simulink model "parallel_prediction_and_cost_function_6phase"  (R2022a)
settings: Solver=FixedStepDiscrete  StartTime=0.0  StopTime=10.0  RelTol=1e-3
undefined symbols (not defined in the file or in its folder): f_c, L_d, L_q, L_x, L_y, p, psi_pm, R_ph
libraries: hdlsllib x5
(part 2 of 3)

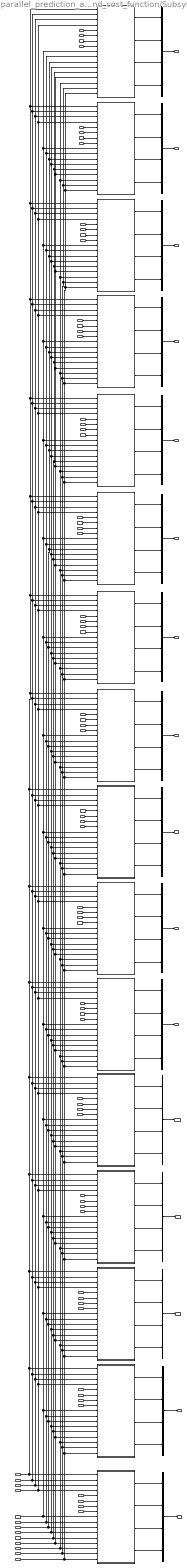
== system parallel_prediction_and_cost_function_6phase/Prediction_and_cost_function/Subsystem ==
  d_phase_voltage_per_switching_state : Inport
  q_phase_voltage_per_switching_state : Inport  Port=2
  x_phase_voltage_per_switching_state : Inport  Port=3
  y_phase_voltage_per_switching_state : Inport  Port=4
  d_phase_voltage_per_switching_state1 : Inport  Port=5
  q_phase_voltage_per_switching_state1 : Inport  Port=6
  x_phase_voltage_per_switching_state1 : Inport  Port=7
  y_phase_voltage_per_switching_state1 : Inport  Port=8
  d_phase_voltage_per_switching_state2 : Inport  Port=9
  q_phase_voltage_per_switching_state2 : Inport  Port=10
  x_phase_voltage_per_switching_state2 : Inport  Port=11
  y_phase_voltage_per_switching_state2 : Inport  Port=12
  d_phase_voltage_per_switching_state3 : Inport  Port=13
  q_phase_voltage_per_switching_state3 : Inport  Port=14
  x_phase_voltage_per_switching_state3 : Inport  Port=15
  y_phase_voltage_per_switching_state3 : Inport  Port=16
  d_phase_voltage_per_switching_state4 : Inport  Port=17
  q_phase_voltage_per_switching_state4 : Inport  Port=18
  x_phase_voltage_per_switching_state4 : Inport  Port=19
  y_phase_voltage_per_switching_state4 : Inport  Port=20
  d_phase_voltage_per_switching_state5 : Inport  Port=21
  q_phase_voltage_per_switching_state5 : Inport  Port=22
  x_phase_voltage_per_switching_state5 : Inport  Port=23
  y_phase_voltage_per_switching_state5 : Inport  Port=24
  d_phase_voltage_per_switching_state6 : Inport  Port=25
  q_phase_voltage_per_switching_state6 : Inport  Port=26
  x_phase_voltage_per_switching_state6 : Inport  Port=27
  y_phase_voltage_per_switching_state6 : Inport  Port=28
  d_phase_voltage_per_switching_state7 : Inport  Port=29
  q_phase_voltage_per_switching_state7 : Inport  Port=30
  x_phase_voltage_per_switching_state7 : Inport  Port=31
  y_phase_voltage_per_switching_state7 : Inport  Port=32
  d_phase_voltage_per_switching_state8 : Inport  Port=33
  q_phase_voltage_per_switching_state8 : Inport  Port=34
  x_phase_voltage_per_switching_state8 : Inport  Port=35
  y_phase_voltage_per_switching_state8 : Inport  Port=36
  d_phase_voltage_per_switching_state9 : Inport  Port=37
  q_phase_voltage_per_switching_state9 : Inport  Port=38
  x_phase_voltage_per_switching_state9 : Inport  Port=39
  y_phase_voltage_per_switching_state9 : Inport  Port=40
  d_phase_voltage_per_switching_state10 : Inport  Port=41
  q_phase_voltage_per_switching_state10 : Inport  Port=42
  x_phase_voltage_per_switching_state10 : Inport  Port=43
  y_phase_voltage_per_switching_state10 : Inport  Port=44
  d_phase_voltage_per_switching_state11 : Inport  Port=45
  q_phase_voltage_per_switching_state11 : Inport  Port=46
  x_phase_voltage_per_switching_state11 : Inport  Port=47
  y_phase_voltage_per_switching_state11 : Inport  Port=48
  d_phase_voltage_per_switching_state12 : Inport  Port=49
  q_phase_voltage_per_switching_state12 : Inport  Port=50
  x_phase_voltage_per_switching_state12 : Inport  Port=51
  y_phase_voltage_per_switching_state12 : Inport  Port=52
  d_phase_voltage_per_switching_state13 : Inport  Port=53
  q_phase_voltage_per_switching_state13 : Inport  Port=54
  x_phase_voltage_per_switching_state13 : Inport  Port=55
  y_phase_voltage_per_switching_state13 : Inport  Port=56
  d_phase_voltage_per_switching_state14 : Inport  Port=57
  q_phase_voltage_per_switching_state14 : Inport  Port=58
  x_phase_voltage_per_switching_state14 : Inport  Port=59
  y_phase_voltage_per_switching_state14 : Inport  Port=60
  SampleTime_div_Ld15 : Inport  Port=61
  SampleTime_div_Lq15 : Inport  Port=62
  SampleTime_div_Lx15 : Inport  Port=63
  SampleTime_div_Ly15 : Inport  Port=64
  id_k_16 : Inport  Port=65
  iq_k_16 : Inport  Port=66
  ix_k_16 : Inport  Port=67
  iy_k_16 : Inport  Port=68
  Rs15 : Inport  Port=69
  omega_el15 : Inport  Port=70
  Lq15 : Inport  Port=71
  Ld15 : Inport  Port=72
  psiPM15 : Inport  Port=73
  d_phase_voltage_per_switching_state15 : Inport  Port=74
  q_phase_voltage_per_switching_state15 : Inport  Port=75
  x_phase_voltage_per_switching_state15 : Inport  Port=76
  y_phase_voltage_per_switching_state15 : Inport  Port=77
  Mux{,1..15} (16 alike) : Mux
  Subsystem : Subsystem
  Subsystem1 : Subsystem
  Subsystem10 : Subsystem
  Subsystem11 : Subsystem
  Subsystem12 : Subsystem
  Subsystem13 : Subsystem
  Subsystem14 : Subsystem
  Subsystem15 : Subsystem
  Subsystem2 : Subsystem
  Subsystem3 : Subsystem
  Subsystem4 : Subsystem
  Subsystem5 : Subsystem
  Subsystem6 : Subsystem
  Subsystem7 : Subsystem
  Subsystem8 : Subsystem
  Subsystem9 : Subsystem
  Prediction_1 : Outport
  Prediction_2 : Outport  Port=2
  Prediction_3 : Outport  Port=3
  Prediction_4 : Outport  Port=4
  Prediction_5 : Outport  Port=5
  Prediction_6 : Outport  Port=6
  Prediction_7 : Outport  Port=7
  Prediction_8 : Outport  Port=8
  Prediction_9 : Outport  Port=9
  Prediction_10 : Outport  Port=10
  Prediction_11 : Outport  Port=11
  Prediction_12 : Outport  Port=12
  Prediction_13 : Outport  Port=13
  Prediction_14 : Outport  Port=14
  Prediction_15 : Outport  Port=15
  Prediction_16 : Outport  Port=16
  wires:
  d_phase_voltage_per_switching_state13/1 -> Subsystem2/5(d_phase_voltage_per_switching_state)
  q_phase_voltage_per_switching_state1/1 -> Subsystem14/6(q_phase_voltage_per_switching_state)
  x_phase_voltage_per_switching_state12/1 -> Subsystem3/7(x_phase_voltage_per_switching_state)
  y_phase_voltage_per_switching_state/1 -> Subsystem15/8(y_phase_voltage_per_switching_state)
  y_phase_voltage_per_switching_state2/1 -> Subsystem13/8(y_phase_voltage_per_switching_state)
  d_phase_voltage_per_switching_state1/1 -> Subsystem14/5(d_phase_voltage_per_switching_state)
  x_phase_voltage_per_switching_state1/1 -> Subsystem14/7(x_phase_voltage_per_switching_state)
  y_phase_voltage_per_switching_state7/1 -> Subsystem8/8(y_phase_voltage_per_switching_state)
  d_phase_voltage_per_switching_state3/1 -> Subsystem12/5(d_phase_voltage_per_switching_state)
  d_phase_voltage_per_switching_state6/1 -> Subsystem9/5(d_phase_voltage_per_switching_state)
  x_phase_voltage_per_switching_state9/1 -> Subsystem6/7(x_phase_voltage_per_switching_state)
  d_phase_voltage_per_switching_state/1 -> Subsystem15/5(d_phase_voltage_per_switching_state)
  x_phase_voltage_per_switching_state3/1 -> Subsystem12/7(x_phase_voltage_per_switching_state)
  d_phase_voltage_per_switching_state2/1 -> Subsystem13/5(d_phase_voltage_per_switching_state)
  x_phase_voltage_per_switching_state8/1 -> Subsystem7/7(x_phase_voltage_per_switching_state)
  y_phase_voltage_per_switching_state9/1 -> Subsystem6/8(y_phase_voltage_per_switching_state)
  x_phase_voltage_per_switching_state4/1 -> Subsystem11/7(x_phase_voltage_per_switching_state)
  y_phase_voltage_per_switching_state1/1 -> Subsystem14/8(y_phase_voltage_per_switching_state)
  q_phase_voltage_per_switching_state2/1 -> Subsystem13/6(q_phase_voltage_per_switching_state)
  x_phase_voltage_per_switching_state2/1 -> Subsystem13/7(x_phase_voltage_per_switching_state)
  y_phase_voltage_per_switching_state11/1 -> Subsystem4/8(y_phase_voltage_per_switching_state)
  y_phase_voltage_per_switching_state4/1 -> Subsystem11/8(y_phase_voltage_per_switching_state)
  x_phase_voltage_per_switching_state/1 -> Subsystem15/7(x_phase_voltage_per_switching_state)
  d_phase_voltage_per_switching_state14/1 -> Subsystem1/5(d_phase_voltage_per_switching_state)
  q_phase_voltage_per_switching_state9/1 -> Subsystem6/6(q_phase_voltage_per_switching_state)
  q_phase_voltage_per_switching_state5/1 -> Subsystem10/6(q_phase_voltage_per_switching_state)
  d_phase_voltage_per_switching_state10/1 -> Subsystem5/5(d_phase_voltage_per_switching_state)
  x_phase_voltage_per_switching_state14/1 -> Subsystem1/7(x_phase_voltage_per_switching_state)
  y_phase_voltage_per_switching_state14/1 -> Subsystem1/8(y_phase_voltage_per_switching_state)
  q_phase_voltage_per_switching_state14/1 -> Subsystem1/6(q_phase_voltage_per_switching_state)
  q_phase_voltage_per_switching_state11/1 -> Subsystem4/6(q_phase_voltage_per_switching_state)
  x_phase_voltage_per_switching_state11/1 -> Subsystem4/7(x_phase_voltage_per_switching_state)
  d_phase_voltage_per_switching_state11/1 -> Subsystem4/5(d_phase_voltage_per_switching_state)
  y_phase_voltage_per_switching_state12/1 -> Subsystem3/8(y_phase_voltage_per_switching_state)
  x_phase_voltage_per_switching_state13/1 -> Subsystem2/7(x_phase_voltage_per_switching_state)
  d_phase_voltage_per_switching_state9/1 -> Subsystem6/5(d_phase_voltage_per_switching_state)
  d_phase_voltage_per_switching_state7/1 -> Subsystem8/5(d_phase_voltage_per_switching_state)
  d_phase_voltage_per_switching_state4/1 -> Subsystem11/5(d_phase_voltage_per_switching_state)
  q_phase_voltage_per_switching_state4/1 -> Subsystem11/6(q_phase_voltage_per_switching_state)
  q_phase_voltage_per_switching_state12/1 -> Subsystem3/6(q_phase_voltage_per_switching_state)
  d_phase_voltage_per_switching_state8/1 -> Subsystem7/5(d_phase_voltage_per_switching_state)
  x_phase_voltage_per_switching_state5/1 -> Subsystem10/7(x_phase_voltage_per_switching_state)
  d_phase_voltage_per_switching_state12/1 -> Subsystem3/5(d_phase_voltage_per_switching_state)
  x_phase_voltage_per_switching_state7/1 -> Subsystem8/7(x_phase_voltage_per_switching_state)
  q_phase_voltage_per_switching_state/1 -> Subsystem15/6(q_phase_voltage_per_switching_state)
  d_phase_voltage_per_switching_state5/1 -> Subsystem10/5(d_phase_voltage_per_switching_state)
  q_phase_voltage_per_switching_state13/1 -> Subsystem2/6(q_phase_voltage_per_switching_state)
  y_phase_voltage_per_switching_state5/1 -> Subsystem10/8(y_phase_voltage_per_switching_state)
  q_phase_voltage_per_switching_state6/1 -> Subsystem9/6(q_phase_voltage_per_switching_state)
  y_phase_voltage_per_switching_state6/1 -> Subsystem9/8(y_phase_voltage_per_switching_state)
  x_phase_voltage_per_switching_state6/1 -> Subsystem9/7(x_phase_voltage_per_switching_state)
  y_phase_voltage_per_switching_state8/1 -> Subsystem7/8(y_phase_voltage_per_switching_state)
  q_phase_voltage_per_switching_state8/1 -> Subsystem7/6(q_phase_voltage_per_switching_state)
  y_phase_voltage_per_switching_state13/1 -> Subsystem2/8(y_phase_voltage_per_switching_state)
  q_phase_voltage_per_switching_state7/1 -> Subsystem8/6(q_phase_voltage_per_switching_state)
  x_phase_voltage_per_switching_state10/1 -> Subsystem5/7(x_phase_voltage_per_switching_state)
  q_phase_voltage_per_switching_state10/1 -> Subsystem5/6(q_phase_voltage_per_switching_state)
  y_phase_voltage_per_switching_state10/1 -> Subsystem5/8(y_phase_voltage_per_switching_state)
  y_phase_voltage_per_switching_state3/1 -> Subsystem12/8(y_phase_voltage_per_switching_state)
  q_phase_voltage_per_switching_state3/1 -> Subsystem12/6(q_phase_voltage_per_switching_state)
  SampleTime_div_Ld15/1 -> Subsystem/1(SampleTime_div_Ld), Subsystem4/1(SampleTime_div_Ld), Subsystem7/1(SampleTime_div_Ld), Subsystem15/1(SampleTime_div_Ld), Subsystem14/1(SampleTime_div_Ld), Subsystem13/1(SampleTime_div_Ld), Subsystem12/1(SampleTime_div_Ld), Subsystem11/1(SampleTime_div_Ld), Subsystem10/1(SampleTime_div_Ld), Subsystem9/1(SampleTime_div_Ld), Subsystem8/1(SampleTime_div_Ld), Subsystem6/1(SampleTime_div_Ld), Subsystem5/1(SampleTime_div_Ld), Subsystem3/1(SampleTime_div_Ld), Subsystem2/1(SampleTime_div_Ld), Subsystem1/1(SampleTime_div_Ld)  "SampleTime_div_Ld"
  SampleTime_div_Lq15/1 -> Subsystem/2(SampleTime_div_Lq), Subsystem4/2(SampleTime_div_Lq), Subsystem15/2(SampleTime_div_Lq), Subsystem14/2(SampleTime_div_Lq), Subsystem13/2(SampleTime_div_Lq), Subsystem12/2(SampleTime_div_Lq), Subsystem11/2(SampleTime_div_Lq), Subsystem10/2(SampleTime_div_Lq), Subsystem9/2(SampleTime_div_Lq), Subsystem8/2(SampleTime_div_Lq), Subsystem7/2(SampleTime_div_Lq), Subsystem6/2(SampleTime_div_Lq), Subsystem5/2(SampleTime_div_Lq), Subsystem3/2(SampleTime_div_Lq), Subsystem2/2(SampleTime_div_Lq), Subsystem1/2(SampleTime_div_Lq)  "SampleTime_div_Lq"
  SampleTime_div_Lx15/1 -> Subsystem/3(SampleTime_div_Lx), Subsystem15/3(SampleTime_div_Lx), Subsystem14/3(SampleTime_div_Lx), Subsystem13/3(SampleTime_div_Lx), Subsystem12/3(SampleTime_div_Lx), Subsystem11/3(SampleTime_div_Lx), Subsystem10/3(SampleTime_div_Lx), Subsystem9/3(SampleTime_div_Lx), Subsystem8/3(SampleTime_div_Lx), Subsystem7/3(SampleTime_div_Lx), Subsystem6/3(SampleTime_div_Lx), Subsystem5/3(SampleTime_div_Lx), Subsystem4/3(SampleTime_div_Lx), Subsystem3/3(SampleTime_div_Lx), Subsystem2/3(SampleTime_div_Lx), Subsystem1/3(SampleTime_div_Lx)  "SampleTime_div_Lx"
  SampleTime_div_Ly15/1 -> Subsystem15/4(SampleTime_div_Ly), Subsystem14/4(SampleTime_div_Ly), Subsystem13/4(SampleTime_div_Ly), Subsystem12/4(SampleTime_div_Ly), Subsystem11/4(SampleTime_div_Ly), Subsystem10/4(SampleTime_div_Ly), Subsystem9/4(SampleTime_div_Ly), Subsystem8/4(SampleTime_div_Ly), Subsystem7/4(SampleTime_div_Ly), Subsystem6/4(SampleTime_div_Ly), Subsystem5/4(SampleTime_div_Ly), Subsystem4/4(SampleTime_div_Ly), Subsystem3/4(SampleTime_div_Ly), Subsystem2/4(SampleTime_div_Ly), Subsystem1/4(SampleTime_div_Ly), Subsystem/4(SampleTime_div_Ly)  "SampleTime_div_Ly"
  d_phase_voltage_per_switching_state15/1 -> Subsystem/5(d_phase_voltage_per_switching_state)
  q_phase_voltage_per_switching_state15/1 -> Subsystem/6(q_phase_voltage_per_switching_state)
  x_phase_voltage_per_switching_state15/1 -> Subsystem/7(x_phase_voltage_per_switching_state)
  y_phase_voltage_per_switching_state15/1 -> Subsystem/8(y_phase_voltage_per_switching_state)
  id_k_16/1 -> Subsystem/9(id_k), Subsystem15/9(id_k), Subsystem14/9(id_k), Subsystem13/9(id_k), Subsystem12/9(id_k), Subsystem11/9(id_k), Subsystem10/9(id_k), Subsystem9/9(id_k), Subsystem8/9(id_k), Subsystem7/9(id_k), Subsystem6/9(id_k), Subsystem5/9(id_k), Subsystem4/9(id_k), Subsystem3/9(id_k), Subsystem2/9(id_k), Subsystem1/9(id_k)  "id_k"
  iq_k_16/1 -> Subsystem/10(iq_k), Subsystem15/10(iq_k), Subsystem14/10(iq_k), Subsystem13/10(iq_k), Subsystem12/10(iq_k), Subsystem11/10(iq_k), Subsystem10/10(iq_k), Subsystem9/10(iq_k), Subsystem8/10(iq_k), Subsystem7/10(iq_k), Subsystem6/10(iq_k), Subsystem5/10(iq_k), Subsystem4/10(iq_k), Subsystem3/10(iq_k), Subsystem2/10(iq_k), Subsystem1/10(iq_k)  "iq_k"
  ix_k_16/1 -> Subsystem/11(ix_k), Subsystem15/11(ix_k), Subsystem14/11(ix_k), Subsystem13/11(ix_k), Subsystem12/11(ix_k), Subsystem11/11(ix_k), Subsystem10/11(ix_k), Subsystem9/11(ix_k), Subsystem8/11(ix_k), Subsystem7/11(ix_k), Subsystem6/11(ix_k), Subsystem5/11(ix_k), Subsystem4/11(ix_k), Subsystem3/11(ix_k), Subsystem2/11(ix_k), Subsystem1/11(ix_k)  "ix_k"
  iy_k_16/1 -> Subsystem/12(iy_k), Subsystem15/12(iy_k), Subsystem14/12(iy_k), Subsystem13/12(iy_k), Subsystem12/12(iy_k), Subsystem11/12(iy_k), Subsystem10/12(iy_k), Subsystem9/12(iy_k), Subsystem8/12(iy_k), Subsystem7/12(iy_k), Subsystem6/12(iy_k), Subsystem5/12(iy_k), Subsystem4/12(iy_k), Subsystem3/12(iy_k), Subsystem2/12(iy_k), Subsystem1/12(iy_k)  "iy_k"
  psiPM15/1 -> Subsystem/13(psiPM), Subsystem10/13(psiPM), Subsystem15/13(psiPM), Subsystem14/13(psiPM), Subsystem13/13(psiPM), Subsystem12/13(psiPM), Subsystem11/13(psiPM), Subsystem9/13(psiPM), Subsystem8/13(psiPM), Subsystem7/13(psiPM), Subsystem6/13(psiPM), Subsystem5/13(psiPM), Subsystem4/13(psiPM), Subsystem3/13(psiPM), Subsystem2/13(psiPM), Subsystem1/13(psiPM)  "psiPM"
  Lq15/1 -> Subsystem/14(Lq), Subsystem15/14(Lq), Subsystem14/14(Lq), Subsystem13/14(Lq), Subsystem12/14(Lq), Subsystem11/14(Lq), Subsystem10/14(Lq), Subsystem9/14(Lq), Subsystem8/14(Lq), Subsystem7/14(Lq), Subsystem6/14(Lq), Subsystem5/14(Lq), Subsystem4/14(Lq), Subsystem3/14(Lq), Subsystem2/14(Lq), Subsystem1/14(Lq)  "Lq"
  Ld15/1 -> Subsystem/15(Ld), Subsystem1/15(Ld), Subsystem15/15(Ld), Subsystem14/15(Ld), Subsystem13/15(Ld), Subsystem12/15(Ld), Subsystem11/15(Ld), Subsystem10/15(Ld), Subsystem9/15(Ld), Subsystem8/15(Ld), Subsystem7/15(Ld), Subsystem6/15(Ld), Subsystem5/15(Ld), Subsystem4/15(Ld), Subsystem3/15(Ld), Subsystem2/15(Ld)  "Ld"
  Rs15/1 -> Subsystem/16(Rs), Subsystem7/16(Rs), Subsystem15/16(Rs), Subsystem14/16(Rs), Subsystem13/16(Rs), Subsystem12/16(Rs), Subsystem11/16(Rs), Subsystem10/16(Rs), Subsystem9/16(Rs), Subsystem8/16(Rs), Subsystem6/16(Rs), Subsystem5/16(Rs), Subsystem4/16(Rs), Subsystem3/16(Rs), Subsystem2/16(Rs), Subsystem1/16(Rs)  "Rs"
  omega_el15/1 -> Subsystem/17(omega_el), Subsystem15/17(omega_el), Subsystem14/17(omega_el), Subsystem13/17(omega_el), Subsystem12/17(omega_el), Subsystem11/17(omega_el), Subsystem10/17(omega_el), Subsystem9/17(omega_el), Subsystem8/17(omega_el), Subsystem7/17(omega_el), Subsystem6/17(omega_el), Subsystem5/17(omega_el), Subsystem4/17(omega_el), Subsystem3/17(omega_el), Subsystem2/17(omega_el), Subsystem1/17(omega_el)  "omega_el"
  Subsystem/4(iy_16) -> Mux/4
  Subsystem/3(ix_16) -> Mux/3
  Subsystem/2(iq_16) -> Mux/2
  Subsystem/1(id_16) -> Mux/1
  Mux/1 -> Prediction_16/1
  Subsystem1/2(iq_15) -> Mux1/2
  Subsystem1/3(ix_15) -> Mux1/3
  Subsystem1/1(id_15) -> Mux1/1
  Mux1/1 -> Prediction_15/1
  Subsystem1/4(iy_15) -> Mux1/4
  Subsystem2/2(iq_14) -> Mux2/2
  Subsystem2/1(id_14) -> Mux2/1
  Subsystem2/3(ix_14) -> Mux2/3
  Subsystem2/4(iy_14) -> Mux2/4
  Mux2/1 -> Prediction_14/1
  Mux3/1 -> Prediction_13/1
  Subsystem3/3(ix_13) -> Mux3/3
  Subsystem3/2(iq_13) -> Mux3/2
  Subsystem3/1(id_13) -> Mux3/1
  Subsystem3/4(iy_13) -> Mux3/4
  Subsystem4/2(iq_12) -> Mux4/2
  Subsystem4/1(id_12) -> Mux4/1
  Mux4/1 -> Prediction_12/1
  Subsystem4/4(iy_12) -> Mux4/4
  Subsystem4/3(ix_12) -> Mux4/3
  Subsystem5/2(iq_11) -> Mux5/2
  Subsystem5/3(ix_11) -> Mux5/3
  Subsystem5/1(id_11) -> Mux5/1
  Subsystem5/4(iy_11) -> Mux5/4
  Mux5/1 -> Prediction_11/1
  Subsystem6/1(id_10) -> Mux6/1
  Subsystem6/2(iq_10) -> Mux6/2
  Subsystem6/3(ix_10) -> Mux6/3
  Subsystem6/4(iy_10) -> Mux6/4
  Mux6/1 -> Prediction_10/1
  Subsystem7/3(ix_9) -> Mux7/3
  Mux7/1 -> Prediction_9/1
  Subsystem7/1(id_9) -> Mux7/1
  Subsystem7/2(iq_9) -> Mux7/2
  Subsystem7/4(iy_9) -> Mux7/4
  Subsystem8/1(id_8) -> Mux8/1
  Subsystem8/3(ix_8) -> Mux8/3
  Subsystem8/2(iq_8) -> Mux8/2
  Subsystem8/4(iy_8) -> Mux8/4
  Mux8/1 -> Prediction_8/1
  Subsystem9/1(id_7) -> Mux9/1
  Subsystem9/3(ix_7) -> Mux9/3
  Subsystem9/4(iy_7) -> Mux9/4
  Subsystem9/2(iq_7) -> Mux9/2
  Mux9/1 -> Prediction_7/1
  Subsystem10/4(iy_6) -> Mux10/4
  Subsystem10/2(iq_6) -> Mux10/2
  Subsystem10/3(ix_6) -> Mux10/3
  Subsystem10/1(id_6) -> Mux10/1
  Mux10/1 -> Prediction_6/1
  Subsystem11/3(ix_5) -> Mux11/3
  Subsystem11/4(iy_5) -> Mux11/4
  Subsystem11/2(iq_5) -> Mux11/2
  Subsystem11/1(id_5) -> Mux11/1
  Mux11/1 -> Prediction_5/1
  Subsystem12/4(iy_4) -> Mux12/4
  Subsystem12/2(iq_4) -> Mux12/2
  Mux12/1 -> Prediction_4/1
  Subsystem12/3(ix_4) -> Mux12/3
  Subsystem12/1(id_4) -> Mux12/1
  Subsystem13/2(iq_3) -> Mux13/2
  Subsystem13/4(iy_3) -> Mux13/4
  Subsystem13/3(ix_3) -> Mux13/3
  Subsystem13/1(id_3) -> Mux13/1
  Mux13/1 -> Prediction_3/1
  Subsystem14/1(id_2) -> Mux14/1
  Subsystem14/3(ix_2) -> Mux14/3
  Subsystem14/2(iq_2) -> Mux14/2
  Subsystem14/4(iy_2) -> Mux14/4
  Mux14/1 -> Prediction_2/1
  Subsystem15/4(iy_1) -> Mux15/4
  Subsystem15/2(iq_1) -> Mux15/2
  Subsystem15/1(id_1) -> Mux15/1
  Subsystem15/3(ix_1) -> Mux15/3
  Mux15/1 -> Prediction_1/1

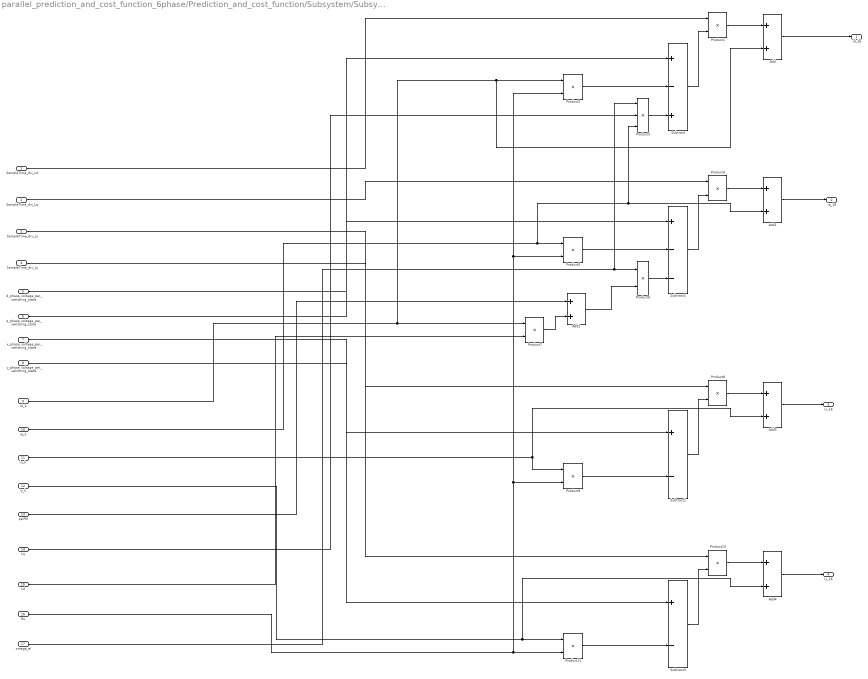
== system parallel_prediction_and_cost_function_6phase/Prediction_and_cost_function/Subsystem/Subsystem ==
  SampleTime_div_Ld : Inport
  SampleTime_div_Lq : Inport  Port=2
  SampleTime_div_Lx : Inport  Port=3
  SampleTime_div_Ly : Inport  Port=4
  d_phase_voltage_per_switching_state : Inport  Port=5
  q_phase_voltage_per_switching_state : Inport  Port=6
  x_phase_voltage_per_switching_state : Inport  Port=7
  y_phase_voltage_per_switching_state : Inport  Port=8
  id_k : Inport  Port=9
  iq_k : Inport  Port=10
  ix_k : Inport  Port=11
  iy_k : Inport  Port=12
  psiPM : Inport  Port=13
  Lq : Inport  Port=14
  Ld : Inport  Port=15
  Rs : Inport  Port=16
  omega_el : Inport  Port=17
  Add{,1,3..4} (4 alike) : Sum  OutDataTypeStr=single
  Add2 : Sum
  Product{1..2,4..11} (10 alike) : Product  OutDataTypeStr=single
  Product3 : Product  Inputs=3  OutDataTypeStr=single
  Subtract : Sum  Inputs=+-+  OutDataTypeStr=single
  Subtract1 : Sum  Inputs=+--  OutDataTypeStr=single
  Subtract2 : Sum  Inputs=+-  OutDataTypeStr=single
  Subtract3 : Sum  Inputs=+-  OutDataTypeStr=single
  id_16 : Outport
  iq_16 : Outport  Port=2
  ix_16 : Outport  Port=3
  iy_16 : Outport  Port=4
  wires:
  q_phase_voltage_per_switching_state/1 -> Subtract1/1
  omega_el/1 -> Product3/1, Product6/1
  Product5/1 -> Subtract1/2
  iq_k/1 -> Product3/3, Add1/2, Product5/1
  iy_k/1 -> Add4/2, Product11/1
  Add2/1 -> Product6/2
  Lq/1 -> Product3/2
  Subtract2/1 -> Product8/2
  SampleTime_div_Ly/1 -> Product10/1
  Rs/1 -> Product9/2, Product2/2, Product5/2, Product11/2
  Product9/1 -> Subtract2/2
  Product8/1 -> Add3/1
  Product7/1 -> Add2/2
  id_k/1 -> Add/2, Product2/1, Product7/1
  x_phase_voltage_per_switching_state/1 -> Subtract2/1
  Product11/1 -> Subtract3/2
  Product6/1 -> Subtract1/3
  Subtract1/1 -> Product4/2
  Product1/1 -> Add/1
  Product10/1 -> Add4/1
  Product4/1 -> Add1/1
  SampleTime_div_Ld/1 -> Product1/1
  y_phase_voltage_per_switching_state/1 -> Subtract3/1
  Product2/1 -> Subtract/2
  Product3/1 -> Subtract/3
  SampleTime_div_Lq/1 -> Product4/1
  Subtract/1 -> Product1/2
  Subtract3/1 -> Product10/2
  psiPM/1 -> Add2/1
  Ld/1 -> Product7/2
  ix_k/1 -> Add3/2, Product9/1
  SampleTime_div_Lx/1 -> Product8/1
  d_phase_voltage_per_switching_state/1 -> Subtract/1
  Add/1 -> id_16/1
  Add1/1 -> iq_16/1
  Add3/1 -> ix_16/1
  Add4/1 -> iy_16/1

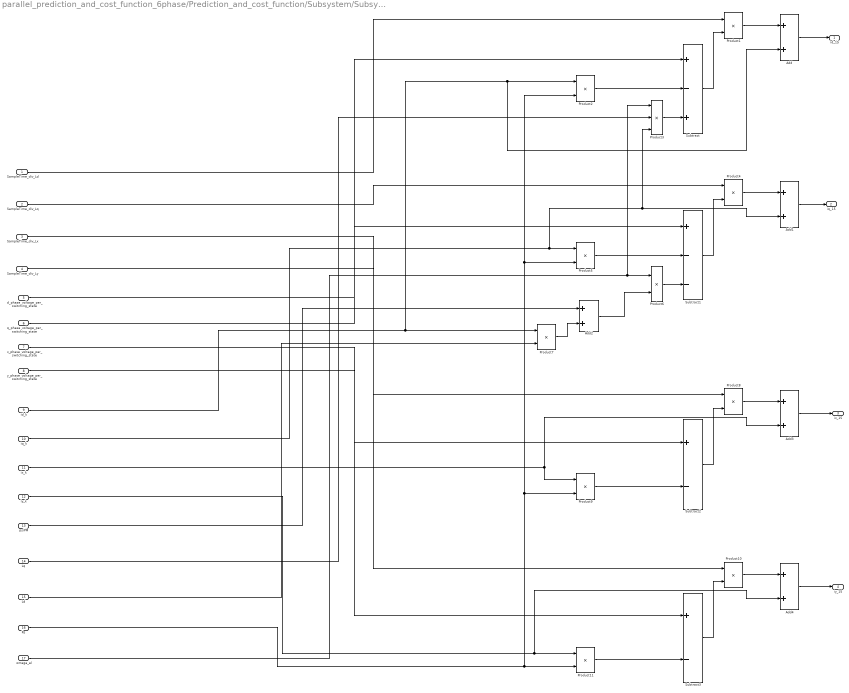
== system parallel_prediction_and_cost_function_6phase/Prediction_and_cost_function/Subsystem/Subsystem1 ==
  SampleTime_div_Ld : Inport
  SampleTime_div_Lq : Inport  Port=2
  SampleTime_div_Lx : Inport  Port=3
  SampleTime_div_Ly : Inport  Port=4
  d_phase_voltage_per_switching_state : Inport  Port=5
  q_phase_voltage_per_switching_state : Inport  Port=6
  x_phase_voltage_per_switching_state : Inport  Port=7
  y_phase_voltage_per_switching_state : Inport  Port=8
  id_k : Inport  Port=9
  iq_k : Inport  Port=10
  ix_k : Inport  Port=11
  iy_k : Inport  Port=12
  psiPM : Inport  Port=13
  Lq : Inport  Port=14
  Ld : Inport  Port=15
  Rs : Inport  Port=16
  omega_el : Inport  Port=17
  Add{,1,3..4} (4 alike) : Sum  OutDataTypeStr=single
  Add2 : Sum
  Product{1..2,4..11} (10 alike) : Product  OutDataTypeStr=single
  Product3 : Product  Inputs=3  OutDataTypeStr=single
  Subtract : Sum  Inputs=+-+  OutDataTypeStr=single
  Subtract1 : Sum  Inputs=+--  OutDataTypeStr=single
  Subtract2 : Sum  Inputs=+-  OutDataTypeStr=single
  Subtract3 : Sum  Inputs=+-  OutDataTypeStr=single
  id_15 : Outport
  iq_15 : Outport  Port=2
  ix_15 : Outport  Port=3
  iy_15 : Outport  Port=4
  wires:
  q_phase_voltage_per_switching_state/1 -> Subtract1/1
  omega_el/1 -> Product3/1, Product6/1
  Product5/1 -> Subtract1/2
  iq_k/1 -> Product3/3, Add1/2, Product5/1
  iy_k/1 -> Add4/2, Product11/1
  Add2/1 -> Product6/2
  Lq/1 -> Product3/2
  Subtract2/1 -> Product8/2
  SampleTime_div_Ly/1 -> Product10/1
  Rs/1 -> Product9/2, Product2/2, Product5/2, Product11/2
  Product9/1 -> Subtract2/2
  Product8/1 -> Add3/1
  Product7/1 -> Add2/2
  id_k/1 -> Add/2, Product2/1, Product7/1
  x_phase_voltage_per_switching_state/1 -> Subtract2/1
  Product11/1 -> Subtract3/2
  Product6/1 -> Subtract1/3
  Subtract1/1 -> Product4/2
  Product1/1 -> Add/1
  Product10/1 -> Add4/1
  Product4/1 -> Add1/1
  SampleTime_div_Ld/1 -> Product1/1
  y_phase_voltage_per_switching_state/1 -> Subtract3/1
  Product2/1 -> Subtract/2
  Product3/1 -> Subtract/3
  SampleTime_div_Lq/1 -> Product4/1
  Subtract/1 -> Product1/2
  Subtract3/1 -> Product10/2
  psiPM/1 -> Add2/1
  Ld/1 -> Product7/2
  ix_k/1 -> Add3/2, Product9/1
  SampleTime_div_Lx/1 -> Product8/1
  d_phase_voltage_per_switching_state/1 -> Subtract/1
  Add/1 -> id_15/1
  Add1/1 -> iq_15/1
  Add3/1 -> ix_15/1
  Add4/1 -> iy_15/1

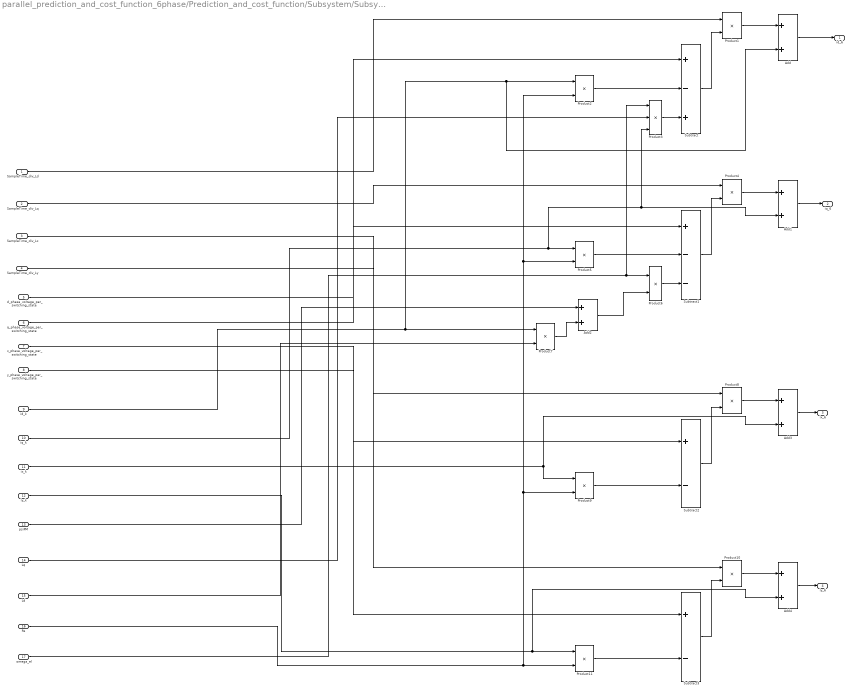
== system parallel_prediction_and_cost_function_6phase/Prediction_and_cost_function/Subsystem/Subsystem10 ==
  SampleTime_div_Ld : Inport
  SampleTime_div_Lq : Inport  Port=2
  SampleTime_div_Lx : Inport  Port=3
  SampleTime_div_Ly : Inport  Port=4
  d_phase_voltage_per_switching_state : Inport  Port=5
  q_phase_voltage_per_switching_state : Inport  Port=6
  x_phase_voltage_per_switching_state : Inport  Port=7
  y_phase_voltage_per_switching_state : Inport  Port=8
  id_k : Inport  Port=9
  iq_k : Inport  Port=10
  ix_k : Inport  Port=11
  iy_k : Inport  Port=12
  psiPM : Inport  Port=13
  Lq : Inport  Port=14
  Ld : Inport  Port=15
  Rs : Inport  Port=16
  omega_el : Inport  Port=17
  Add{,1,3..4} (4 alike) : Sum  OutDataTypeStr=single
  Add2 : Sum
  Product{1..2,4..11} (10 alike) : Product  OutDataTypeStr=single
  Product3 : Product  Inputs=3  OutDataTypeStr=single
  Subtract : Sum  Inputs=+-+  OutDataTypeStr=single
  Subtract1 : Sum  Inputs=+--  OutDataTypeStr=single
  Subtract2 : Sum  Inputs=+-  OutDataTypeStr=single
  Subtract3 : Sum  Inputs=+-  OutDataTypeStr=single
  id_6 : Outport
  iq_6 : Outport  Port=2
  ix_6 : Outport  Port=3
  iy_6 : Outport  Port=4
  wires:
  q_phase_voltage_per_switching_state/1 -> Subtract1/1
  omega_el/1 -> Product3/1, Product6/1
  Product5/1 -> Subtract1/2
  iq_k/1 -> Product3/3, Add1/2, Product5/1
  iy_k/1 -> Add4/2, Product11/1
  Add2/1 -> Product6/2
  Lq/1 -> Product3/2
  Subtract2/1 -> Product8/2
  SampleTime_div_Ly/1 -> Product10/1
  Rs/1 -> Product9/2, Product2/2, Product5/2, Product11/2
  Product9/1 -> Subtract2/2
  Product8/1 -> Add3/1
  Product7/1 -> Add2/2
  id_k/1 -> Add/2, Product2/1, Product7/1
  x_phase_voltage_per_switching_state/1 -> Subtract2/1
  Product11/1 -> Subtract3/2
  Product6/1 -> Subtract1/3
  Subtract1/1 -> Product4/2
  Product1/1 -> Add/1
  Product10/1 -> Add4/1
  Product4/1 -> Add1/1
  SampleTime_div_Ld/1 -> Product1/1
  y_phase_voltage_per_switching_state/1 -> Subtract3/1
  Product2/1 -> Subtract/2
  Product3/1 -> Subtract/3
  SampleTime_div_Lq/1 -> Product4/1
  Subtract/1 -> Product1/2
  Subtract3/1 -> Product10/2
  psiPM/1 -> Add2/1
  Ld/1 -> Product7/2
  ix_k/1 -> Add3/2, Product9/1
  SampleTime_div_Lx/1 -> Product8/1
  d_phase_voltage_per_switching_state/1 -> Subtract/1
  Add/1 -> id_6/1
  Add1/1 -> iq_6/1
  Add3/1 -> ix_6/1
  Add4/1 -> iy_6/1

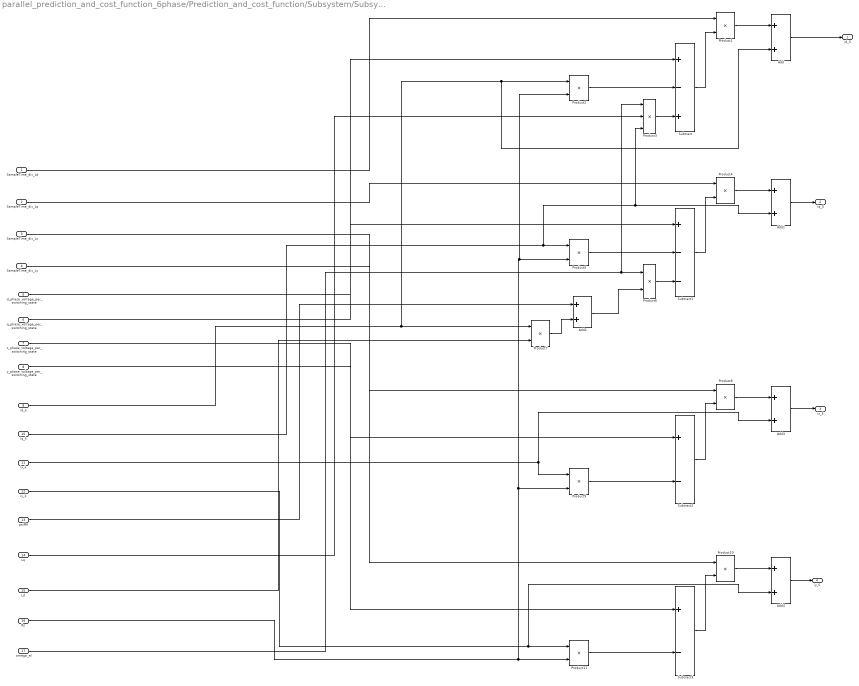
== system parallel_prediction_and_cost_function_6phase/Prediction_and_cost_function/Subsystem/Subsystem11 ==
  SampleTime_div_Ld : Inport
  SampleTime_div_Lq : Inport  Port=2
  SampleTime_div_Lx : Inport  Port=3
  SampleTime_div_Ly : Inport  Port=4
  d_phase_voltage_per_switching_state : Inport  Port=5
  q_phase_voltage_per_switching_state : Inport  Port=6
  x_phase_voltage_per_switching_state : Inport  Port=7
  y_phase_voltage_per_switching_state : Inport  Port=8
  id_k : Inport  Port=9
  iq_k : Inport  Port=10
  ix_k : Inport  Port=11
  iy_k : Inport  Port=12
  psiPM : Inport  Port=13
  Lq : Inport  Port=14
  Ld : Inport  Port=15
  Rs : Inport  Port=16
  omega_el : Inport  Port=17
  Add{,1,3..4} (4 alike) : Sum  OutDataTypeStr=single
  Add2 : Sum
  Product{1..2,4..11} (10 alike) : Product  OutDataTypeStr=single
  Product3 : Product  Inputs=3  OutDataTypeStr=single
  Subtract : Sum  Inputs=+-+  OutDataTypeStr=single
  Subtract1 : Sum  Inputs=+--  OutDataTypeStr=single
  Subtract2 : Sum  Inputs=+-  OutDataTypeStr=single
  Subtract3 : Sum  Inputs=+-  OutDataTypeStr=single
  id_5 : Outport
  iq_5 : Outport  Port=2
  ix_5 : Outport  Port=3
  iy_5 : Outport  Port=4
  wires:
  q_phase_voltage_per_switching_state/1 -> Subtract1/1
  omega_el/1 -> Product3/1, Product6/1
  Product5/1 -> Subtract1/2
  iq_k/1 -> Product3/3, Add1/2, Product5/1
  iy_k/1 -> Add4/2, Product11/1
  Add2/1 -> Product6/2
  Lq/1 -> Product3/2
  Subtract2/1 -> Product8/2
  SampleTime_div_Ly/1 -> Product10/1
  Rs/1 -> Product9/2, Product2/2, Product5/2, Product11/2
  Product9/1 -> Subtract2/2
  Product8/1 -> Add3/1
  Product7/1 -> Add2/2
  id_k/1 -> Add/2, Product2/1, Product7/1
  x_phase_voltage_per_switching_state/1 -> Subtract2/1
  Product11/1 -> Subtract3/2
  Product6/1 -> Subtract1/3
  Subtract1/1 -> Product4/2
  Product1/1 -> Add/1
  Product10/1 -> Add4/1
  Product4/1 -> Add1/1
  SampleTime_div_Ld/1 -> Product1/1
  y_phase_voltage_per_switching_state/1 -> Subtract3/1
  Product2/1 -> Subtract/2
  Product3/1 -> Subtract/3
  SampleTime_div_Lq/1 -> Product4/1
  Subtract/1 -> Product1/2
  Subtract3/1 -> Product10/2
  psiPM/1 -> Add2/1
  Ld/1 -> Product7/2
  ix_k/1 -> Add3/2, Product9/1
  SampleTime_div_Lx/1 -> Product8/1
  d_phase_voltage_per_switching_state/1 -> Subtract/1
  Add/1 -> id_5/1
  Add1/1 -> iq_5/1
  Add3/1 -> ix_5/1
  Add4/1 -> iy_5/1

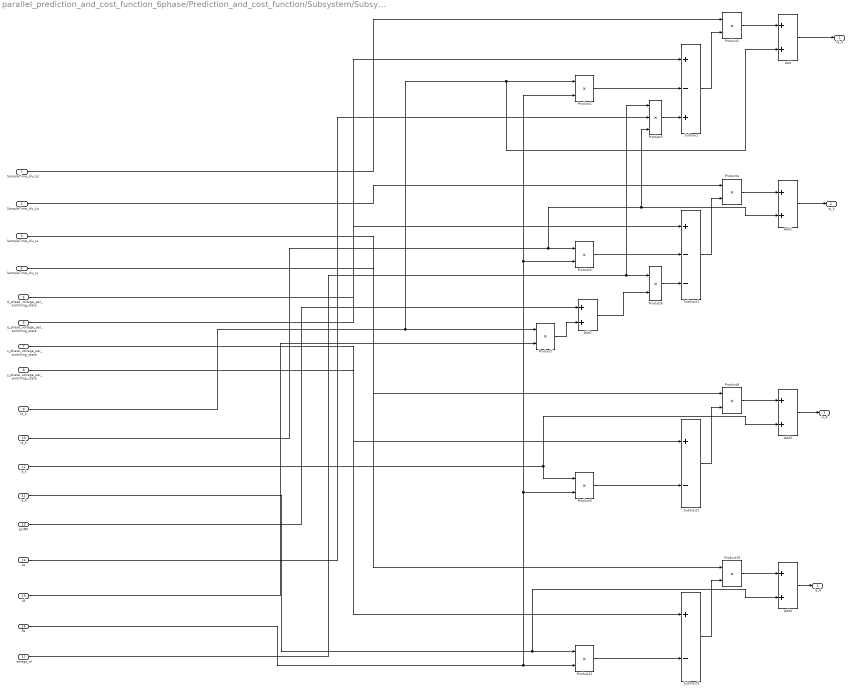
== system parallel_prediction_and_cost_function_6phase/Prediction_and_cost_function/Subsystem/Subsystem12 ==
  SampleTime_div_Ld : Inport
  SampleTime_div_Lq : Inport  Port=2
  SampleTime_div_Lx : Inport  Port=3
  SampleTime_div_Ly : Inport  Port=4
  d_phase_voltage_per_switching_state : Inport  Port=5
  q_phase_voltage_per_switching_state : Inport  Port=6
  x_phase_voltage_per_switching_state : Inport  Port=7
  y_phase_voltage_per_switching_state : Inport  Port=8
  id_k : Inport  Port=9
  iq_k : Inport  Port=10
  ix_k : Inport  Port=11
  iy_k : Inport  Port=12
  psiPM : Inport  Port=13
  Lq : Inport  Port=14
  Ld : Inport  Port=15
  Rs : Inport  Port=16
  omega_el : Inport  Port=17
  Add{,1,3..4} (4 alike) : Sum  OutDataTypeStr=single
  Add2 : Sum
  Product{1..2,4..11} (10 alike) : Product  OutDataTypeStr=single
  Product3 : Product  Inputs=3  OutDataTypeStr=single
  Subtract : Sum  Inputs=+-+  OutDataTypeStr=single
  Subtract1 : Sum  Inputs=+--  OutDataTypeStr=single
  Subtract2 : Sum  Inputs=+-  OutDataTypeStr=single
  Subtract3 : Sum  Inputs=+-  OutDataTypeStr=single
  id_4 : Outport
  iq_4 : Outport  Port=2
  ix_4 : Outport  Port=3
  iy_4 : Outport  Port=4
  wires:
  q_phase_voltage_per_switching_state/1 -> Subtract1/1
  omega_el/1 -> Product3/1, Product6/1
  Product5/1 -> Subtract1/2
  iq_k/1 -> Product3/3, Add1/2, Product5/1
  iy_k/1 -> Add4/2, Product11/1
  Add2/1 -> Product6/2
  Lq/1 -> Product3/2
  Subtract2/1 -> Product8/2
  SampleTime_div_Ly/1 -> Product10/1
  Rs/1 -> Product9/2, Product2/2, Product5/2, Product11/2
  Product9/1 -> Subtract2/2
  Product8/1 -> Add3/1
  Product7/1 -> Add2/2
  id_k/1 -> Add/2, Product2/1, Product7/1
  x_phase_voltage_per_switching_state/1 -> Subtract2/1
  Product11/1 -> Subtract3/2
  Product6/1 -> Subtract1/3
  Subtract1/1 -> Product4/2
  Product1/1 -> Add/1
  Product10/1 -> Add4/1
  Product4/1 -> Add1/1
  SampleTime_div_Ld/1 -> Product1/1
  y_phase_voltage_per_switching_state/1 -> Subtract3/1
  Product2/1 -> Subtract/2
  Product3/1 -> Subtract/3
  SampleTime_div_Lq/1 -> Product4/1
  Subtract/1 -> Product1/2
  Subtract3/1 -> Product10/2
  psiPM/1 -> Add2/1
  Ld/1 -> Product7/2
  ix_k/1 -> Add3/2, Product9/1
  SampleTime_div_Lx/1 -> Product8/1
  d_phase_voltage_per_switching_state/1 -> Subtract/1
  Add/1 -> id_4/1
  Add1/1 -> iq_4/1
  Add3/1 -> ix_4/1
  Add4/1 -> iy_4/1

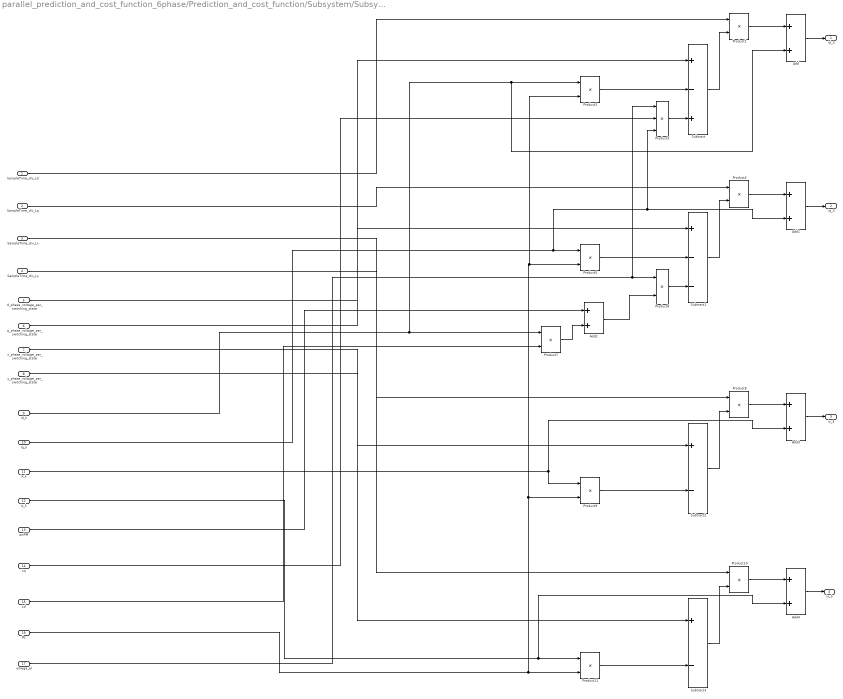
== system parallel_prediction_and_cost_function_6phase/Prediction_and_cost_function/Subsystem/Subsystem13 ==
  SampleTime_div_Ld : Inport
  SampleTime_div_Lq : Inport  Port=2
  SampleTime_div_Lx : Inport  Port=3
  SampleTime_div_Ly : Inport  Port=4
  d_phase_voltage_per_switching_state : Inport  Port=5
  q_phase_voltage_per_switching_state : Inport  Port=6
  x_phase_voltage_per_switching_state : Inport  Port=7
  y_phase_voltage_per_switching_state : Inport  Port=8
  id_k : Inport  Port=9
  iq_k : Inport  Port=10
  ix_k : Inport  Port=11
  iy_k : Inport  Port=12
  psiPM : Inport  Port=13
  Lq : Inport  Port=14
  Ld : Inport  Port=15
  Rs : Inport  Port=16
  omega_el : Inport  Port=17
  Add{,1,3..4} (4 alike) : Sum  OutDataTypeStr=single
  Add2 : Sum
  Product{1..2,4..11} (10 alike) : Product  OutDataTypeStr=single
  Product3 : Product  Inputs=3  OutDataTypeStr=single
  Subtract : Sum  Inputs=+-+  OutDataTypeStr=single
  Subtract1 : Sum  Inputs=+--  OutDataTypeStr=single
  Subtract2 : Sum  Inputs=+-  OutDataTypeStr=single
  Subtract3 : Sum  Inputs=+-  OutDataTypeStr=single
  id_3 : Outport
  iq_3 : Outport  Port=2
  ix_3 : Outport  Port=3
  iy_3 : Outport  Port=4
  wires:
  q_phase_voltage_per_switching_state/1 -> Subtract1/1
  omega_el/1 -> Product3/1, Product6/1
  Product5/1 -> Subtract1/2
  iq_k/1 -> Product3/3, Add1/2, Product5/1
  iy_k/1 -> Add4/2, Product11/1
  Add2/1 -> Product6/2
  Lq/1 -> Product3/2
  Subtract2/1 -> Product8/2
  SampleTime_div_Ly/1 -> Product10/1
  Rs/1 -> Product9/2, Product2/2, Product5/2, Product11/2
  Product9/1 -> Subtract2/2
  Product8/1 -> Add3/1
  Product7/1 -> Add2/2
  id_k/1 -> Add/2, Product2/1, Product7/1
  x_phase_voltage_per_switching_state/1 -> Subtract2/1
  Product11/1 -> Subtract3/2
  Product6/1 -> Subtract1/3
  Subtract1/1 -> Product4/2
  Product1/1 -> Add/1
  Product10/1 -> Add4/1
  Product4/1 -> Add1/1
  SampleTime_div_Ld/1 -> Product1/1
  y_phase_voltage_per_switching_state/1 -> Subtract3/1
  Product2/1 -> Subtract/2
  Product3/1 -> Subtract/3
  SampleTime_div_Lq/1 -> Product4/1
  Subtract/1 -> Product1/2
  Subtract3/1 -> Product10/2
  psiPM/1 -> Add2/1
  Ld/1 -> Product7/2
  ix_k/1 -> Add3/2, Product9/1
  SampleTime_div_Lx/1 -> Product8/1
  d_phase_voltage_per_switching_state/1 -> Subtract/1
  Add/1 -> id_3/1
  Add1/1 -> iq_3/1
  Add3/1 -> ix_3/1
  Add4/1 -> iy_3/1

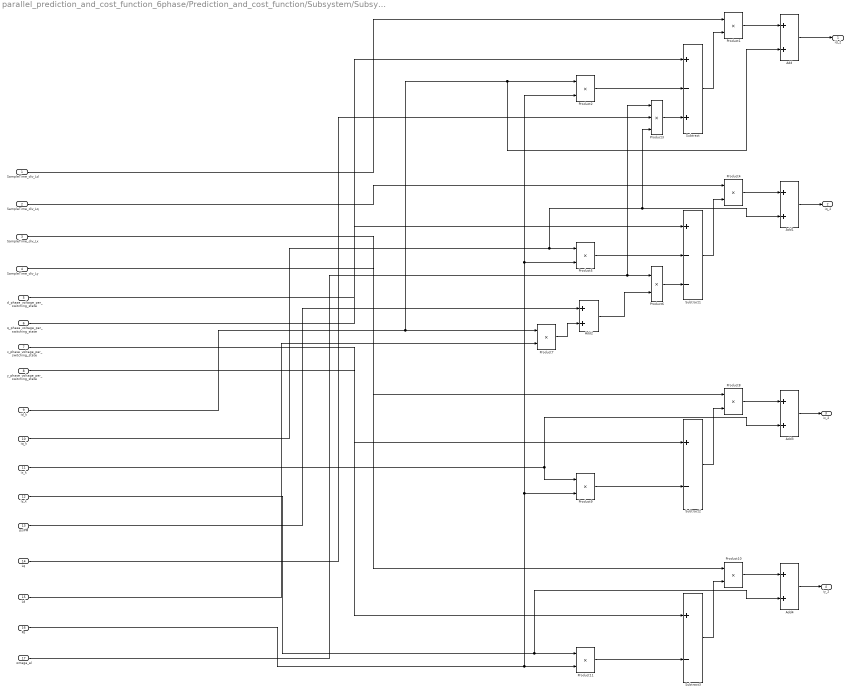
== system parallel_prediction_and_cost_function_6phase/Prediction_and_cost_function/Subsystem/Subsystem14 ==
  SampleTime_div_Ld : Inport
  SampleTime_div_Lq : Inport  Port=2
  SampleTime_div_Lx : Inport  Port=3
  SampleTime_div_Ly : Inport  Port=4
  d_phase_voltage_per_switching_state : Inport  Port=5
  q_phase_voltage_per_switching_state : Inport  Port=6
  x_phase_voltage_per_switching_state : Inport  Port=7
  y_phase_voltage_per_switching_state : Inport  Port=8
  id_k : Inport  Port=9
  iq_k : Inport  Port=10
  ix_k : Inport  Port=11
  iy_k : Inport  Port=12
  psiPM : Inport  Port=13
  Lq : Inport  Port=14
  Ld : Inport  Port=15
  Rs : Inport  Port=16
  omega_el : Inport  Port=17
  Add{,1,3..4} (4 alike) : Sum  OutDataTypeStr=single
  Add2 : Sum
  Product{1..2,4..11} (10 alike) : Product  OutDataTypeStr=single
  Product3 : Product  Inputs=3  OutDataTypeStr=single
  Subtract : Sum  Inputs=+-+  OutDataTypeStr=single
  Subtract1 : Sum  Inputs=+--  OutDataTypeStr=single
  Subtract2 : Sum  Inputs=+-  OutDataTypeStr=single
  Subtract3 : Sum  Inputs=+-  OutDataTypeStr=single
  id_2 : Outport
  iq_2 : Outport  Port=2
  ix_2 : Outport  Port=3
  iy_2 : Outport  Port=4
  wires:
  q_phase_voltage_per_switching_state/1 -> Subtract1/1
  omega_el/1 -> Product3/1, Product6/1
  Product5/1 -> Subtract1/2
  iq_k/1 -> Product3/3, Add1/2, Product5/1
  iy_k/1 -> Add4/2, Product11/1
  Add2/1 -> Product6/2
  Lq/1 -> Product3/2
  Subtract2/1 -> Product8/2
  SampleTime_div_Ly/1 -> Product10/1
  Rs/1 -> Product9/2, Product2/2, Product5/2, Product11/2
  Product9/1 -> Subtract2/2
  Product8/1 -> Add3/1
  Product7/1 -> Add2/2
  id_k/1 -> Add/2, Product2/1, Product7/1
  x_phase_voltage_per_switching_state/1 -> Subtract2/1
  Product11/1 -> Subtract3/2
  Product6/1 -> Subtract1/3
  Subtract1/1 -> Product4/2
  Product1/1 -> Add/1
  Product10/1 -> Add4/1
  Product4/1 -> Add1/1
  SampleTime_div_Ld/1 -> Product1/1
  y_phase_voltage_per_switching_state/1 -> Subtract3/1
  Product2/1 -> Subtract/2
  Product3/1 -> Subtract/3
  SampleTime_div_Lq/1 -> Product4/1
  Subtract/1 -> Product1/2
  Subtract3/1 -> Product10/2
  psiPM/1 -> Add2/1
  Ld/1 -> Product7/2
  ix_k/1 -> Add3/2, Product9/1
  SampleTime_div_Lx/1 -> Product8/1
  d_phase_voltage_per_switching_state/1 -> Subtract/1
  Add/1 -> id_2/1
  Add1/1 -> iq_2/1
  Add3/1 -> ix_2/1
  Add4/1 -> iy_2/1

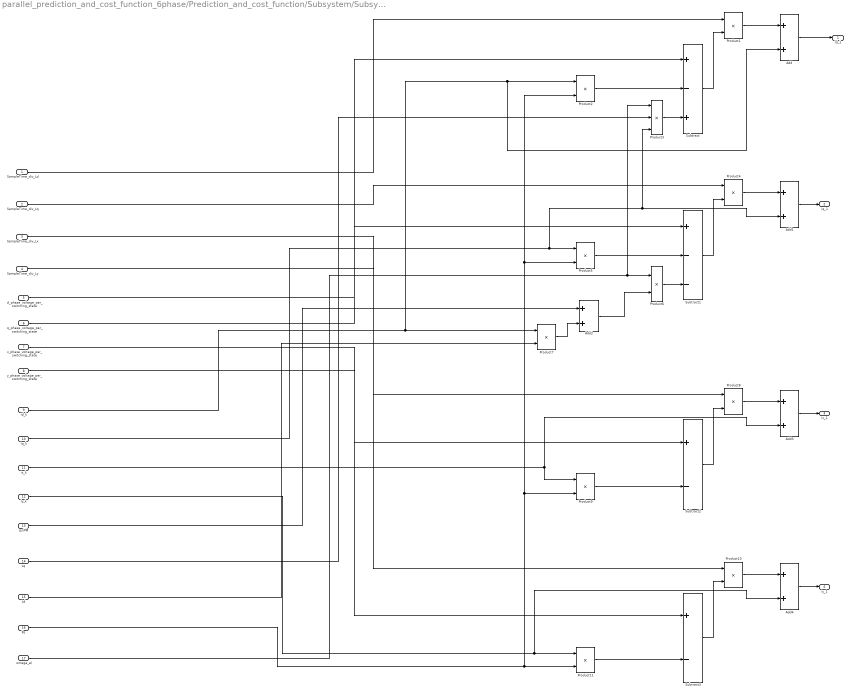
== system parallel_prediction_and_cost_function_6phase/Prediction_and_cost_function/Subsystem/Subsystem15 ==
  SampleTime_div_Ld : Inport
  SampleTime_div_Lq : Inport  Port=2
  SampleTime_div_Lx : Inport  Port=3
  SampleTime_div_Ly : Inport  Port=4
  d_phase_voltage_per_switching_state : Inport  Port=5
  q_phase_voltage_per_switching_state : Inport  Port=6
  x_phase_voltage_per_switching_state : Inport  Port=7
  y_phase_voltage_per_switching_state : Inport  Port=8
  id_k : Inport  Port=9
  iq_k : Inport  Port=10
  ix_k : Inport  Port=11
  iy_k : Inport  Port=12
  psiPM : Inport  Port=13
  Lq : Inport  Port=14
  Ld : Inport  Port=15
  Rs : Inport  Port=16
  omega_el : Inport  Port=17
  Add{,1,3..4} (4 alike) : Sum  OutDataTypeStr=single
  Add2 : Sum
  Product{1..2,4..11} (10 alike) : Product  OutDataTypeStr=single
  Product3 : Product  Inputs=3  OutDataTypeStr=single
  Subtract : Sum  Inputs=+-+  OutDataTypeStr=single
  Subtract1 : Sum  Inputs=+--  OutDataTypeStr=single
  Subtract2 : Sum  Inputs=+-  OutDataTypeStr=single
  Subtract3 : Sum  Inputs=+-  OutDataTypeStr=single
  id_1 : Outport
  iq_1 : Outport  Port=2
  ix_1 : Outport  Port=3
  iy_1 : Outport  Port=4
  wires:
  q_phase_voltage_per_switching_state/1 -> Subtract1/1
  omega_el/1 -> Product3/1, Product6/1
  Product5/1 -> Subtract1/2
  iq_k/1 -> Product3/3, Add1/2, Product5/1
  iy_k/1 -> Add4/2, Product11/1
  Add2/1 -> Product6/2
  Lq/1 -> Product3/2
  Subtract2/1 -> Product8/2
  SampleTime_div_Ly/1 -> Product10/1
  Rs/1 -> Product9/2, Product2/2, Product5/2, Product11/2
  Product9/1 -> Subtract2/2
  Product8/1 -> Add3/1
  Product7/1 -> Add2/2
  id_k/1 -> Add/2, Product2/1, Product7/1
  x_phase_voltage_per_switching_state/1 -> Subtract2/1
  Product11/1 -> Subtract3/2
  Product6/1 -> Subtract1/3
  Subtract1/1 -> Product4/2
  Product1/1 -> Add/1
  Product10/1 -> Add4/1
  Product4/1 -> Add1/1
  SampleTime_div_Ld/1 -> Product1/1
  y_phase_voltage_per_switching_state/1 -> Subtract3/1
  Product2/1 -> Subtract/2
  Product3/1 -> Subtract/3
  SampleTime_div_Lq/1 -> Product4/1
  Subtract/1 -> Product1/2
  Subtract3/1 -> Product10/2
  psiPM/1 -> Add2/1
  Ld/1 -> Product7/2
  ix_k/1 -> Add3/2, Product9/1
  SampleTime_div_Lx/1 -> Product8/1
  d_phase_voltage_per_switching_state/1 -> Subtract/1
  Add/1 -> id_1/1
  Add1/1 -> iq_1/1
  Add3/1 -> ix_1/1
  Add4/1 -> iy_1/1

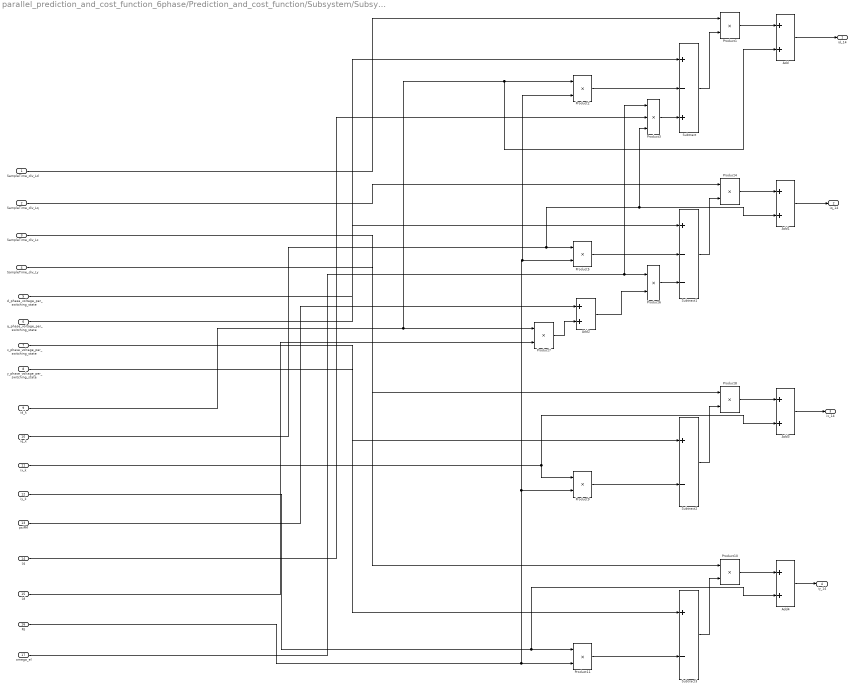
== system parallel_prediction_and_cost_function_6phase/Prediction_and_cost_function/Subsystem/Subsystem2 ==
  SampleTime_div_Ld : Inport
  SampleTime_div_Lq : Inport  Port=2
  SampleTime_div_Lx : Inport  Port=3
  SampleTime_div_Ly : Inport  Port=4
  d_phase_voltage_per_switching_state : Inport  Port=5
  q_phase_voltage_per_switching_state : Inport  Port=6
  x_phase_voltage_per_switching_state : Inport  Port=7
  y_phase_voltage_per_switching_state : Inport  Port=8
  id_k : Inport  Port=9
  iq_k : Inport  Port=10
  ix_k : Inport  Port=11
  iy_k : Inport  Port=12
  psiPM : Inport  Port=13
  Lq : Inport  Port=14
  Ld : Inport  Port=15
  Rs : Inport  Port=16
  omega_el : Inport  Port=17
  Add{,1,3..4} (4 alike) : Sum  OutDataTypeStr=single
  Add2 : Sum
  Product{1..2,4..11} (10 alike) : Product  OutDataTypeStr=single
  Product3 : Product  Inputs=3  OutDataTypeStr=single
  Subtract : Sum  Inputs=+-+  OutDataTypeStr=single
  Subtract1 : Sum  Inputs=+--  OutDataTypeStr=single
  Subtract2 : Sum  Inputs=+-  OutDataTypeStr=single
  Subtract3 : Sum  Inputs=+-  OutDataTypeStr=single
  id_14 : Outport
  iq_14 : Outport  Port=2
  ix_14 : Outport  Port=3
  iy_14 : Outport  Port=4
  wires:
  q_phase_voltage_per_switching_state/1 -> Subtract1/1
  omega_el/1 -> Product3/1, Product6/1
  Product5/1 -> Subtract1/2
  iq_k/1 -> Product3/3, Add1/2, Product5/1
  iy_k/1 -> Add4/2, Product11/1
  Add2/1 -> Product6/2
  Lq/1 -> Product3/2
  Subtract2/1 -> Product8/2
  SampleTime_div_Ly/1 -> Product10/1
  Rs/1 -> Product9/2, Product2/2, Product5/2, Product11/2
  Product9/1 -> Subtract2/2
  Product8/1 -> Add3/1
  Product7/1 -> Add2/2
  id_k/1 -> Add/2, Product2/1, Product7/1
  x_phase_voltage_per_switching_state/1 -> Subtract2/1
  Product11/1 -> Subtract3/2
  Product6/1 -> Subtract1/3
  Subtract1/1 -> Product4/2
  Product1/1 -> Add/1
  Product10/1 -> Add4/1
  Product4/1 -> Add1/1
  SampleTime_div_Ld/1 -> Product1/1
  y_phase_voltage_per_switching_state/1 -> Subtract3/1
  Product2/1 -> Subtract/2
  Product3/1 -> Subtract/3
  SampleTime_div_Lq/1 -> Product4/1
  Subtract/1 -> Product1/2
  Subtract3/1 -> Product10/2
  psiPM/1 -> Add2/1
  Ld/1 -> Product7/2
  ix_k/1 -> Add3/2, Product9/1
  SampleTime_div_Lx/1 -> Product8/1
  d_phase_voltage_per_switching_state/1 -> Subtract/1
  Add/1 -> id_14/1
  Add1/1 -> iq_14/1
  Add3/1 -> ix_14/1
  Add4/1 -> iy_14/1

== system parallel_prediction_and_cost_function_6phase/Prediction_and_cost_function/Subsystem/Subsystem3 ==
  SampleTime_div_Ld : Inport
  SampleTime_div_Lq : Inport  Port=2
  SampleTime_div_Lx : Inport  Port=3
  SampleTime_div_Ly : Inport  Port=4
  d_phase_voltage_per_switching_state : Inport  Port=5
  q_phase_voltage_per_switching_state : Inport  Port=6
  x_phase_voltage_per_switching_state : Inport  Port=7
  y_phase_voltage_per_switching_state : Inport  Port=8
  id_k : Inport  Port=9
  iq_k : Inport  Port=10
  ix_k : Inport  Port=11
  iy_k : Inport  Port=12
  psiPM : Inport  Port=13
  Lq : Inport  Port=14
  Ld : Inport  Port=15
  Rs : Inport  Port=16
  omega_el : Inport  Port=17
  Add{,1,3..4} (4 alike) : Sum  OutDataTypeStr=single
  Add2 : Sum
  Product{1..2,4..11} (10 alike) : Product  OutDataTypeStr=single
  Product3 : Product  Inputs=3  OutDataTypeStr=single
  Subtract : Sum  Inputs=+-+  OutDataTypeStr=single
  Subtract1 : Sum  Inputs=+--  OutDataTypeStr=single
  Subtract2 : Sum  Inputs=+-  OutDataTypeStr=single
  Subtract3 : Sum  Inputs=+-  OutDataTypeStr=single
  id_13 : Outport
  iq_13 : Outport  Port=2
  ix_13 : Outport  Port=3
  iy_13 : Outport  Port=4
  wires:
  q_phase_voltage_per_switching_state/1 -> Subtract1/1
  omega_el/1 -> Product3/1, Product6/1
  Product5/1 -> Subtract1/2
  iq_k/1 -> Product3/3, Add1/2, Product5/1
  iy_k/1 -> Add4/2, Product11/1
  Add2/1 -> Product6/2
  Lq/1 -> Product3/2
  Subtract2/1 -> Product8/2
  SampleTime_div_Ly/1 -> Product10/1
  Rs/1 -> Product9/2, Product2/2, Product5/2, Product11/2
  Product9/1 -> Subtract2/2
  Product8/1 -> Add3/1
  Product7/1 -> Add2/2
  id_k/1 -> Add/2, Product2/1, Product7/1
  x_phase_voltage_per_switching_state/1 -> Subtract2/1
  Product11/1 -> Subtract3/2
  Product6/1 -> Subtract1/3
  Subtract1/1 -> Product4/2
  Product1/1 -> Add/1
  Product10/1 -> Add4/1
  Product4/1 -> Add1/1
  SampleTime_div_Ld/1 -> Product1/1
  y_phase_voltage_per_switching_state/1 -> Subtract3/1
  Product2/1 -> Subtract/2
  Product3/1 -> Subtract/3
  SampleTime_div_Lq/1 -> Product4/1
  Subtract/1 -> Product1/2
  Subtract3/1 -> Product10/2
  psiPM/1 -> Add2/1
  Ld/1 -> Product7/2
  ix_k/1 -> Add3/2, Product9/1
  SampleTime_div_Lx/1 -> Product8/1
  d_phase_voltage_per_switching_state/1 -> Subtract/1
  Add/1 -> id_13/1
  Add1/1 -> iq_13/1
  Add3/1 -> ix_13/1
  Add4/1 -> iy_13/1

== system parallel_prediction_and_cost_function_6phase/Prediction_and_cost_function/Subsystem/Subsystem4 ==
  SampleTime_div_Ld : Inport
  SampleTime_div_Lq : Inport  Port=2
  SampleTime_div_Lx : Inport  Port=3
  SampleTime_div_Ly : Inport  Port=4
  d_phase_voltage_per_switching_state : Inport  Port=5
  q_phase_voltage_per_switching_state : Inport  Port=6
  x_phase_voltage_per_switching_state : Inport  Port=7
  y_phase_voltage_per_switching_state : Inport  Port=8
  id_k : Inport  Port=9
  iq_k : Inport  Port=10
  ix_k : Inport  Port=11
  iy_k : Inport  Port=12
  psiPM : Inport  Port=13
  Lq : Inport  Port=14
  Ld : Inport  Port=15
  Rs : Inport  Port=16
  omega_el : Inport  Port=17
  Add{,1,3..4} (4 alike) : Sum  OutDataTypeStr=single
  Add2 : Sum
  Product{1..2,4..11} (10 alike) : Product  OutDataTypeStr=single
  Product3 : Product  Inputs=3  OutDataTypeStr=single
  Subtract : Sum  Inputs=+-+  OutDataTypeStr=single
  Subtract1 : Sum  Inputs=+--  OutDataTypeStr=single
  Subtract2 : Sum  Inputs=+-  OutDataTypeStr=single
  Subtract3 : Sum  Inputs=+-  OutDataTypeStr=single
  id_12 : Outport
  iq_12 : Outport  Port=2
  ix_12 : Outport  Port=3
  iy_12 : Outport  Port=4
  wires:
  q_phase_voltage_per_switching_state/1 -> Subtract1/1
  omega_el/1 -> Product3/1, Product6/1
  Product5/1 -> Subtract1/2
  iq_k/1 -> Product3/3, Add1/2, Product5/1
  iy_k/1 -> Add4/2, Product11/1
  Add2/1 -> Product6/2
  Lq/1 -> Product3/2
  Subtract2/1 -> Product8/2
  SampleTime_div_Ly/1 -> Product10/1
  Rs/1 -> Product9/2, Product2/2, Product5/2, Product11/2
  Product9/1 -> Subtract2/2
  Product8/1 -> Add3/1
  Product7/1 -> Add2/2
  id_k/1 -> Add/2, Product2/1, Product7/1
  x_phase_voltage_per_switching_state/1 -> Subtract2/1
  Product11/1 -> Subtract3/2
  Product6/1 -> Subtract1/3
  Subtract1/1 -> Product4/2
  Product1/1 -> Add/1
  Product10/1 -> Add4/1
  Product4/1 -> Add1/1
  SampleTime_div_Ld/1 -> Product1/1
  y_phase_voltage_per_switching_state/1 -> Subtract3/1
  Product2/1 -> Subtract/2
  Product3/1 -> Subtract/3
  SampleTime_div_Lq/1 -> Product4/1
  Subtract/1 -> Product1/2
  Subtract3/1 -> Product10/2
  psiPM/1 -> Add2/1
  Ld/1 -> Product7/2
  ix_k/1 -> Add3/2, Product9/1
  SampleTime_div_Lx/1 -> Product8/1
  d_phase_voltage_per_switching_state/1 -> Subtract/1
  Add/1 -> id_12/1
  Add1/1 -> iq_12/1
  Add3/1 -> ix_12/1
  Add4/1 -> iy_12/1

== system parallel_prediction_and_cost_function_6phase/Prediction_and_cost_function/Subsystem/Subsystem5 ==
  SampleTime_div_Ld : Inport
  SampleTime_div_Lq : Inport  Port=2
  SampleTime_div_Lx : Inport  Port=3
  SampleTime_div_Ly : Inport  Port=4
  d_phase_voltage_per_switching_state : Inport  Port=5
  q_phase_voltage_per_switching_state : Inport  Port=6
  x_phase_voltage_per_switching_state : Inport  Port=7
  y_phase_voltage_per_switching_state : Inport  Port=8
  id_k : Inport  Port=9
  iq_k : Inport  Port=10
  ix_k : Inport  Port=11
  iy_k : Inport  Port=12
  psiPM : Inport  Port=13
  Lq : Inport  Port=14
  Ld : Inport  Port=15
  Rs : Inport  Port=16
  omega_el : Inport  Port=17
  Add{,1,3..4} (4 alike) : Sum  OutDataTypeStr=single
  Add2 : Sum
  Product{1..2,4..11} (10 alike) : Product  OutDataTypeStr=single
  Product3 : Product  Inputs=3  OutDataTypeStr=single
  Subtract : Sum  Inputs=+-+  OutDataTypeStr=single
  Subtract1 : Sum  Inputs=+--  OutDataTypeStr=single
  Subtract2 : Sum  Inputs=+-  OutDataTypeStr=single
  Subtract3 : Sum  Inputs=+-  OutDataTypeStr=single
  id_11 : Outport
  iq_11 : Outport  Port=2
  ix_11 : Outport  Port=3
  iy_11 : Outport  Port=4
  wires:
  q_phase_voltage_per_switching_state/1 -> Subtract1/1
  omega_el/1 -> Product3/1, Product6/1
  Product5/1 -> Subtract1/2
  iq_k/1 -> Product3/3, Add1/2, Product5/1
  iy_k/1 -> Add4/2, Product11/1
  Add2/1 -> Product6/2
  Lq/1 -> Product3/2
  Subtract2/1 -> Product8/2
  SampleTime_div_Ly/1 -> Product10/1
  Rs/1 -> Product9/2, Product2/2, Product5/2, Product11/2
  Product9/1 -> Subtract2/2
  Product8/1 -> Add3/1
  Product7/1 -> Add2/2
  id_k/1 -> Add/2, Product2/1, Product7/1
  x_phase_voltage_per_switching_state/1 -> Subtract2/1
  Product11/1 -> Subtract3/2
  Product6/1 -> Subtract1/3
  Subtract1/1 -> Product4/2
  Product1/1 -> Add/1
  Product10/1 -> Add4/1
  Product4/1 -> Add1/1
  SampleTime_div_Ld/1 -> Product1/1
  y_phase_voltage_per_switching_state/1 -> Subtract3/1
  Product2/1 -> Subtract/2
  Product3/1 -> Subtract/3
  SampleTime_div_Lq/1 -> Product4/1
  Subtract/1 -> Product1/2
  Subtract3/1 -> Product10/2
  psiPM/1 -> Add2/1
  Ld/1 -> Product7/2
  ix_k/1 -> Add3/2, Product9/1
  SampleTime_div_Lx/1 -> Product8/1
  d_phase_voltage_per_switching_state/1 -> Subtract/1
  Add/1 -> id_11/1
  Add1/1 -> iq_11/1
  Add3/1 -> ix_11/1
  Add4/1 -> iy_11/1
